simulink model "Maglev_FeedbackLin"  (R2025a)
settings: Solver=ode4  StartTime=0.0  StopTime=T_sim  FixedStep=1e-4  RelTol=1e-6  AbsTol=1e-8
PreLoadFcn:
  | % Modellpfad abrufen
  | modelPath = fileparts(which(bdroot));
  | projectRoot = fileparts(modelPath);
  | 
  | % Simulationsumgebung einrichten und Parameter laden
  | run(fullfile(projectRoot, 'setup_sim_params.m'));
  | load(fullfile(projectRoot, 'Controller_Params', 'EKFData.mat'));
  | load(fullfile(projectRoot, 'Controller_Params', 'NonlinearControllerData.mat'));
undefined symbols (not defined in the file): ekf_params, Ext_Fina_Val, Ext_Init_Val, grav, I_max, I_min, Km, mass, Plant, T_stp
libraries: fl_lib x11, nesl_utility x4
settings Model: Creator=Meng Lingbing  LastModifiedBy=CelestialAurora
settings SolverCC: AutoScaleAbsTol=off  MaxConsecutiveMinStep=10  AlgebraicLoopSolver=TrustRegion  AutoInsertRateTranBlk=on  MaxZcPerStep=1.0
settings DebuggingCC: AlgebraicLoopMsg=none  UnconnectedInputMsg=warning  UnconnectedOutputMsg=warning  UnconnectedLineMsg=warning  SymbolicDimsDataTypeCodeGenerationDiagnostic=none
settings ModelReferenceCC: EnableRefExpFcnMdlSchedulingChecks=on
settings SFSimCC: CustomCodeUndefinedFunction=UseInterfaceOnly
settings RTWCC: GPUComputeCapability=3.5  DLArmComputeVersion=19.05
settings SimscapeCC: ExplicitSolverDiagnosticOptions=none  SimscapeLogType=all  SimscapeLogSimulationStatistics=on  SimscapeLogDataHistory=10000.0

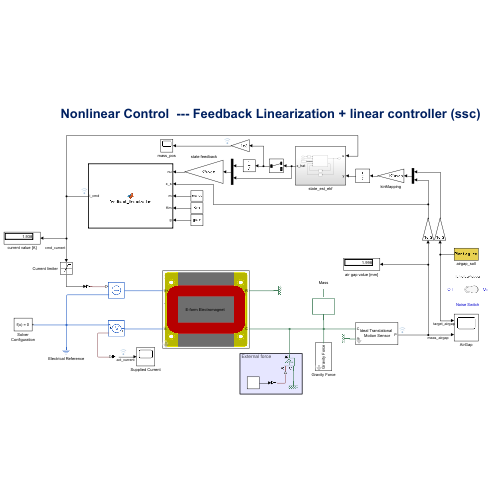
[thumbnail: Simulink's stored preview of the top-level diagram]
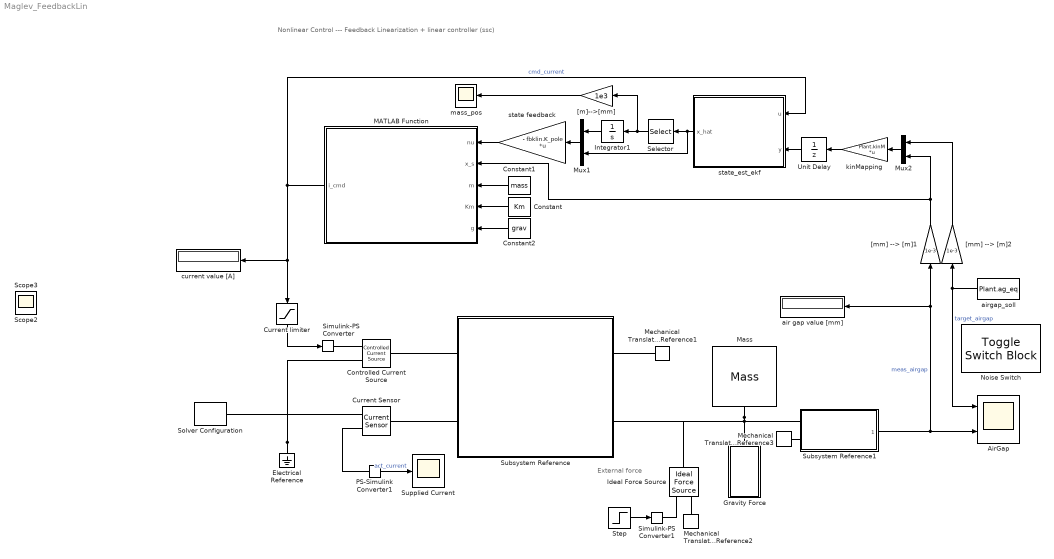
== system Maglev_FeedbackLin ==
  note: Nonlinear Control --- Feedback Linearization + linear controller (ssc)
  note: External force
  AirGap : Scope  NumInputPorts=2
      settings: ActiveDisplayYMinimum=1.7984458962721404  ActiveDisplayYMaximum=2.5832142457823677
  Constant : Constant  Value=Km
  Constant1 : Constant  Value=mass
  Constant2 : Constant  Value=grav
  Controlled Current Source : fl_lib/Electrical/Electrical Sources/Controlled Current Source
  Current Sensor : fl_lib/Electrical/Electrical Sensors/Current Sensor
  Current limiter : Saturate  UpperLimit=I_max  LowerLimit=I_min
  Electrical Reference : fl_lib/Electrical/Electrical Elements/Electrical Reference
  Gravity Force : Subsystem
      mask DialogControl DescGroupVar Prompt: Gravity Force
      mask DialogControl DescTextVar Prompt: Fg = Mass*grav, as constant parameters predefined
      mask DialogControl DescTextVar2 Prompt: Direction: Downward
      mask Display: disp("Gravity Force")
  Ideal Force Source : fl_lib/Mechanical/Mechanical Sources/Ideal Force Source
  Integrator1 : Integrator
  MATLAB Function : MATLAB Function  TreatAsAtomicUnit=on
  Mass : fl_lib/Mechanical/Translational Elements/Mass  mass=mass kg  num_ports=foundation.enum.numPorts2.one  v_specify=on  v_priority=Low  v=0 m/s  v_nominal_specify=off  v_nominal_value=1  v_nominal_unit=m/s  f_specify=off  f_priority=None  f=0 N  f_nominal_specify=off  f_nominal_value=700  f_nominal_unit=N
  Mechanical Translational Reference1 : fl_lib/Mechanical/Translational Elements/Mechanical Translational Reference
  Mechanical Translational Reference2 : fl_lib/Mechanical/Translational Elements/Mechanical Translational Reference
  Mechanical Translational Reference3 : fl_lib/Mechanical/Translational Elements/Mechanical Translational Reference
  Mux1 : Mux  Inputs=2
  Mux2 : Mux  Inputs=2
  Noise Switch : ToggleSwitchBlock
  PS-Simulink Converter1 : nesl_utility/PS-Simulink Converter  PhysicalDomain=network_engine_domain  SubClassName=ps_output  LeftPortType=input  RightPortType=output  PseudoPeriodic=off  Frequencies=[]  VectorFormat=inherit  Unit=inherit  AffineConversion=off
  Selector : Selector  InputPortWidth=2  IndexOptions=Index vector (dialog)  Indices=[1]  OutputSizes=1
  Simulink-PS Converter : nesl_utility/Simulink-PS Converter  PhysicalDomain=network_engine_domain  SubClassName=ps_input  LeftPortType=input  RightPortType=output  PseudoPeriodic=off  Frequencies=[]  NoiseDistribution=none  NoiseParameters=[]  Unit=1  AffineConversion=off  FilteringAndDerivatives=zero  SimscapeFilterOrder=1  InputFilterTimeConstant=0.001  UdotUserProvided=0
  Simulink-PS Converter1 : nesl_utility/Simulink-PS Converter  PhysicalDomain=network_engine_domain  SubClassName=ps_input  LeftPortType=input  RightPortType=output  PseudoPeriodic=off  Frequencies=[]  NoiseDistribution=none  NoiseParameters=[]  Unit=1  AffineConversion=off  FilteringAndDerivatives=filter  SimscapeFilterOrder=1  InputFilterTimeConstant=0.001  UdotUserProvided=0
  Solver Configuration : nesl_utility/Solver Configuration  PhysicalDomain=network_engine_domain  SubClassName=solver  LeftPortType=input  RightPortType=generic  Tones=[]  Harmonics=[]  SimulateNoise=off  Profile=off  UseLocalSampling=off  EnableSwitchedLinearOptims=on  FrequencyDomain=off  UseCCode=off  RelTol=0.001  AbsTol=1e-06  MinStep=1e-09  ToWorkspace=off  RevertToSquareIcSolve=off  NumHomotopyIterations=100  PhasorMode=off  PhasorModeNumHarmonics=1  ConsistencySolver=NEWTON_XTOL_AFTER_FTOL  IndexReductionMethod=DerivativeReplacement  DoDC=off  ResidualTolerance=1e-09  ConsistencyTolSource=GLOBAL  ConsistencyAbsTol=0.001  ConsistencyRelTol=0.001  ConsistencyTolFactor=0.001  UseLocalSolver=off  LocalSolverChoice=NE_BACKWARD_EULER_ADVANCER  ResolveIndetEquations=on  FunctionEvalNumThread=1  LocalSolverSampleTime=0.001  DoFixedCost=off  MaxNonlinIter=3  MaxModeIter=2  ComputeImpulses=off  ImpulseIterations=2  LinearAlgebra=auto  LinearAlgebraNumThread=0  EquationFormulation=NE_TIME_EF  DelaysMemoryBudget=1024  AutomaticFiltering=on  FilteringTimeConstant=0.001  PartitionStorageMethod=AS_NEEDED  PartitionMemoryBudget=1024  PartitionMethod=ROBUST  MultibodyUseLocalSolver=off  MultibodyLocalSolverChoice=ODE1  MultibodyLocalSolverSampleTime=0.001
  Step : Step  Time=T_stp  Before=Ext_Init_Val  After=Ext_Fina_Val  SampleTime=0
  Subsystem Reference : Subsystem  ReferencedSubsystem=IntegratedElectromagnet  l_airgap=airgap_init
  Subsystem Reference1 : Subsystem  ReferencedSubsystem=IdealTrans_MotionSensor  ns_sw=isNoiseActive  ns_pw=NoisePower  ts=Ts  init_pos=airgap_init
  Supplied Current : Scope
      settings: ActiveDisplayYMinimum=-0.44982538634132796  ActiveDisplayYMaximum=8.7852856748355368  DataLoggingVariableName=ScopeData3
  Unit Delay : UnitDelay  InitialCondition=Plant.x_init(1)  SampleTime=-1  HasFrameUpgradeWarning=on
  "[m]-->[mm]" : Gain  Gain=1e3
  "[mm] --> [m]1" : Gain  Gain=1e-3
  "[mm] --> [m]2" : Gain  Gain=1e-3
  air gap value [mm] : Display
      settings: Decimation=4
  airgap_soll : Constant  Value=Plant.ag_eq
  current value [A] : Display
  kinMapping : Gain  Gain=Plant.kinM  Multiplication=Matrix(K*u) (u vector)
  mass_pos : Scope
      settings: ActiveDisplayYMinimum=-0.61234907793782922  ActiveDisplayYMaximum=0.21389745350689768  DataLoggingVariableName=ScopeData4
  state feedback : Gain  Gain=- fbklin.K_pole  Multiplication=Matrix(K*u) (u vector)
  state_est_ekf : Subsystem
  Scope2 : Scope
      settings: ActiveDisplayYMinimum=2.68786  ActiveDisplayYMaximum=51.73117
  Scope3 : Scope
      settings: ActiveDisplayYMinimum=-19475.53313  ActiveDisplayYMaximum=27959.62036  DataLoggingVariableName=ScopeData2
  wires:
  Current limiter/1 -> Simulink-PS Converter/1
  PS-Simulink Converter1/1 -> Supplied Current/1  "act_current"
  Step/1 -> Simulink-PS Converter1/1
  Constant/1 -> MATLAB Function/4(Km)
  Constant1/1 -> MATLAB Function/3(m)
  Constant2/1 -> MATLAB Function/5(g)
  Subsystem Reference1/1 -> air gap value [mm]/1, "[mm] --> [m]1"/1, AirGap/2  "meas_airgap"
  Mux1/1 -> state feedback/1
  state feedback/1 -> MATLAB Function/1(nu)
  MATLAB Function/1(i_cmd) -> state_est_ekf/1(u), Current limiter/1, current value [A]/1  "cmd_current"
  Mux2/1 -> kinMapping/1
  "[m]-->[mm]"/1 -> mass_pos/1
  Selector/1 -> "[m]-->[mm]"/1, Integrator1/1
  Unit Delay/1 -> state_est_ekf/2(y)
  kinMapping/1 -> Unit Delay/1
  Integrator1/1 -> Mux1/1
  state_est_ekf/1(x_hat) -> Selector/1, Mux1/2
  "[mm] --> [m]1"/1 -> MATLAB Function/2(x_s), Mux2/2
  airgap_soll/1 -> "[mm] --> [m]2"/1, AirGap/1  "target_airgap"
  "[mm] --> [m]2"/1 -> Mux2/1
  connections:
  Electrical Reference/LConn1 -- Current Sensor/RConn2 -- Controlled Current Source/RConn2 -- Solver Configuration/RConn1
  Mass/LConn1 -- Subsystem Reference1/LConn1 -- Gravity Force/RConn1 -- Subsystem Reference/RConn2 -- Ideal Force Source/LConn1
  Subsystem Reference/RConn1 -- Mechanical Translational Reference1/LConn1
  Simulink-PS Converter/RConn1 -- Controlled Current Source/RConn1
  Subsystem Reference/LConn2 -- Current Sensor/LConn1
  PS-Simulink Converter1/LConn1 -- Current Sensor/RConn1
  Subsystem Reference/LConn1 -- Controlled Current Source/LConn1
  Simulink-PS Converter1/RConn1 -- Ideal Force Source/RConn1
  Mechanical Translational Reference2/LConn1 -- Ideal Force Source/RConn2
  Mechanical Translational Reference3/LConn1 -- Subsystem Reference1/LConn2

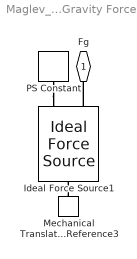
== system Maglev_FeedbackLin/Gravity Force ==
  Ideal Force Source1 : fl_lib/Mechanical/Mechanical Sources/Ideal Force Source
  Mechanical Translational Reference3 : fl_lib/Mechanical/Translational Elements/Mechanical Translational Reference
  PS Constant : fl_lib/Physical Signals/Sources/PS Constant  constant=mass*grav N
  Fg : PMIOPort  Side=Right
  connections:
  Mechanical Translational Reference3/LConn1 -- Ideal Force Source1/LConn1
  PS Constant/RConn1 -- Ideal Force Source1/RConn1
  Ideal Force Source1/RConn2 -- Fg/RConn1

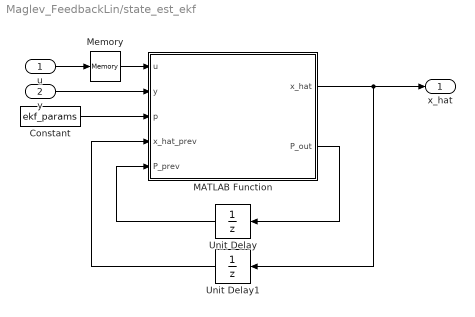
== system Maglev_FeedbackLin/state_est_ekf ==
  u : Inport
  y : Inport  Port=2
  Constant : Constant  Value=ekf_params  OutDataTypeStr=Bus: ekf_Bus
  MATLAB Function : MATLAB Function  TreatAsAtomicUnit=on
  Memory : Memory  InitialCondition=ekf_params.u0
  Unit Delay : UnitDelay  InitialCondition=ekf_params.P0  SampleTime=-1  HasFrameUpgradeWarning=on
  Unit Delay1 : UnitDelay  InitialCondition=ekf_params.x0  SampleTime=-1  HasFrameUpgradeWarning=on
  x_hat : Outport
  wires:
  MATLAB Function/2(P_out) -> Unit Delay/1
  MATLAB Function/1(x_hat) -> x_hat/1, Unit Delay1/1
  Constant/1 -> MATLAB Function/3(p)
  Unit Delay1/1 -> MATLAB Function/4(x_hat_prev)
  Unit Delay/1 -> MATLAB Function/5(P_prev)
  y/1 -> MATLAB Function/2(y)
  u/1 -> Memory/1
  Memory/1 -> MATLAB Function/1(u)

== matlab function Maglev_FeedbackLin/state_est_ekf/MATLAB Function ==
  data: u input; y input; p input; x_hat output; x_hat_prev input; P_prev input; P_out output
function [x_hat, P_out] = ekf_maglev(u, y, p, x_hat_prev, P_prev)
    % EKF for single-magnet levitation system
    %
    % Inputs:
    %   y           - measured position deviation x1 (scalar, with noise)
    %   u           - applied current i_s (scalar, control input)
    %   x_hat_prev  - state estimate from previous step [x1_hat; x2_hat]
    %   P_prev      - covariance from previous step (2x2)
    %   Km, m, g    - plant parameters
    %   x0          - nominal air gap (2e-3 m)
    %   Ts          - sample period
    %   Q           - process noise covariance (2x2, design parameter)
    %   R           - measurement noise covariance (scalar, sensor spec)
    %
    % Outputs:
    %   x_hat       - updated state estimate [x1_hat; x2_hat]
    %   P_out       - updated covariance (2x2)
    
    Ts = p.Ts;  Q = p.Q;  R = p.R;  H = p.H;
    Km = p.Km;  m = p.m;  g = p.g;  x0 = p.x_gap;

    %% --- 1. Predict step ---
    % Evaluate nonlinear dynamics at previous estimate
    x1 = x_hat_prev(1);
    x2 = x_hat_prev(2);
    
    % Guard against numerical issues if estimate drifts toward magnet
    gap = max(x0 - x1, 1e-9);
    
    % Predicted state (Euler integration of nonlinear dynamics)
    x_pred = [ x1 + Ts * x2;
               x2 + Ts * ( (Km/m) * u^2 / gap^2 - g ) ];
    
    % Jacobian F evaluated at previous estimate
    F = [ 1,                                    Ts;
          Ts * 2 * Km * u^2 / (m * gap^3),       1  ];
    
    % Predicted covariance
    P_pred = F * P_prev * F' + Q;
    
    %% --- 2. Update step ---
    % H = [1, 0];                  % measure position only
    
    % Innovation
    y_pred = H * x_pred;
    innov  = y - y_pred;
    
    % Innovation covariance
    S = H * P_pred * H' + R;
    
    % Kalman gain
    K = (P_pred * H') / S;
    
    % Corrected state and covariance
    x_hat = x_pred + K * innov;
    P_out = (eye(2) - K * H) * P_pred;
    
    % Symmetrize to fight numerical drift
    P_out = 0.5 * (P_out + P_out');
end

== matlab function Maglev_FeedbackLin/MATLAB Function ==
  data: nu input; x_s input; m input; i_cmd output; Km input; g input
function i_cmd = feedback_linearization(nu, x_s, m, Km, g)
% INPUT-OUTPUT FEEDBACK LINEARIZATION

% Inputs:
%   x_s   : measured actual air gap (m)
%   nu    : virtual input from outer linear controller (m/s²)
%   m     : mass of the slide (kg)
%   Km    : magnetic force constant (N·m²/A²)
%   g     : gravity (m/s²)
%
% Output:
%   i_cmd   : commanded coil current (A)

    epsilon = 1e-10;   % safety margin to avoid division by zero / negative sqrt
    
    % Saturate air gap (never let it reach zero)
    xs_sat = max(x_s, epsilon);
    
    % prevent negative argument (anti-windup effect)
    nu_sat  = max(nu, -g + 0.05);        % soft limit

    % Compute argument of square root
    arg = (m / Km) * (nu_sat + g);
    
    % Positive root only + saturation
    i_cmd = xs_sat * sqrt(max(arg, 0));
end
